simulink model "Optical_Movement_Detection_PAR"  (Simulink 7.5)
settings: Solver=ode45  StartTime=0.0  StopTime=inf  RelTol=1e-3
values from neighbouring files (symbols this model uses):
  D = 1    [Copter_Animation.m]
  HSE_Bottom_1 = imresize(imread('D:\GoogleMapsBilder\PAR\HSE_Bottom_1.jpg'), 1)    [TESTS_Optical_Flow_Scenarios.m]
undefined symbols (not defined in the file or in its folder): fspecial, Kanade, Low, Lucas, Rec, SDTV
libraries: simulink x13, dspobslib x10, vipgeotforms x3, vipanalysis x3, dspstat3 x3, dspmtrx3 x2, dspsigops x2, vipconversions x1, dspswit3 x1, vipsrcs x1, viptextngfix x1, vipsnks x1
(part 1 of 2)
settings Model: Creator=roczit00  LastModifiedBy=Anonymos
settings DataIOCC: SaveOutput=off  DSMLogging=off  SaveTime=off
settings DebuggingCC: AlgebraicLoopMsg=none  SolverPrmCheckMsg=none  UnconnectedInputMsg=none  UnconnectedOutputMsg=none  UnconnectedLineMsg=none  StrictBusMsg=Warning

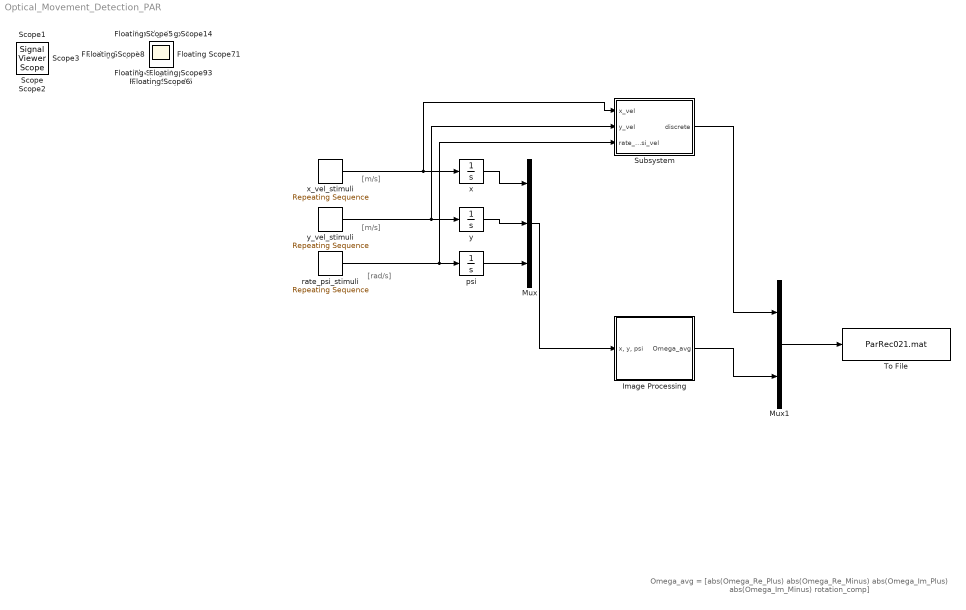
== system Optical_Movement_Detection_PAR ==
  note: [m/s]
  note: [m/s]
  note: [rad/s]
  note: Omega_avg = [abs(Omega_Re_Plus) abs(Omega_Re_Minus) abs(Omega_Im_Plus) abs(Omega_Im_Minus) rotation_comp]
  Image Processing : Subsystem  mask{Ts_Opt=10, Cam_Img_Dim=[100,100], Env_Orig=[2144 1424], Block_Matching_Size=[31,31], Block_Matching_Overlap=[0 0], Block_Matching_Max_Disp=[7 7], Omega_avg_Gain=1/1000, load_cmd=HSE_Bottom_1}
      mask prompts: Ts_Opt "Camera's frames per second (1/SampleTime):"; Cam_Img_Dim "Cameras size of the synthetic image [R C]:"; Env_Orig "Initial image center of environment [R C]:"; Block_Matching_Size "Block size of optical flow block matching algorithm [heigh width]"; Block_Matching_Overlap "Block Overlap [R C] :"; Block_Matching_Max_Disp "Maximum displacement [R C]:"; Omega_avg_Gain "Gain of detected velocity vector"; load_cmd "Load Cmd"
      mask init:
      | set_param(gcb,'MaskSelfModifiable','on')
      mask TabNameString: General,General,General,Block Matching,Block Matching,Block Matching,Block Matching,General
  Mux : Mux  Inputs=3
  Mux1 : Mux  Inputs=2
  Subsystem : Subsystem  mask{In_Val_Sample_Time=0.01}
      mask prompts: In_Val_Sample_Time "Sample time"
  To File : ToFile  Filename=ParRec021.mat  MatrixName=Tfile
  psi : Integrator
  rate_psi_stimuli : simulink/Sources/Repeating Sequence  SystemSampleTime=-1  rep_seq_t=[0,10]  rep_seq_y=[0,0]
  x : Integrator
  x_vel_stimuli : simulink/Sources/Repeating Sequence  SystemSampleTime=-1  rep_seq_t=[0,1]  rep_seq_y=[0,0.5]
  y : Integrator
  y_vel_stimuli : simulink/Sources/Repeating Sequence  SystemSampleTime=-1  rep_seq_t=[0,10]  rep_seq_y=[0,0]
  Floating Scope{,1..15} (16 alike) : Scope
      Floating Scope settings: Floating=on  YMin=-40  YMax=90
      Floating Scope1 settings: Floating=on
      Floating Scope10 settings: Floating=on  SaveName=ScopeData12
      Floating Scope11 settings: Floating=on  SaveName=ScopeData13
      Floating Scope12 settings: Floating=on  YMin=-2500  YMax=27500  SaveName=ScopeData14
      Floating Scope13 settings: Floating=on  YMin=3  YMax=7  SaveName=ScopeData15
      Floating Scope14 settings: Floating=on  SaveName=ScopeData16
      Floating Scope15 settings: Floating=on  SaveName=ScopeData17
      Floating Scope2 settings: Floating=on  YMin=-6000  YMax=2500  SaveName=ScopeData2
      Floating Scope3 settings: Floating=on  SaveName=ScopeData3
      Floating Scope4 settings: Floating=on  SaveName=ScopeData4
      Floating Scope5 settings: Floating=on  YMin=-0.7  YMax=0.8  SaveName=ScopeData5
      Floating Scope6 settings: Floating=on  YMin=-1  YMax=1  SaveName=ScopeData6
      Floating Scope7 settings: Floating=on  YMin=-15  YMax=10  SaveName=ScopeData7
      Floating Scope8 settings: Floating=on  YMax=45  SaveName=ScopeData10
      Floating Scope9 settings: Floating=on  YMin=-7  YMax=9  SaveName=ScopeData11
  Scope{,1..3} (4 alike) : SignalViewerScope  IOType=viewer  RefreshTime=0.035000
      Scope settings: YMin=-0.01  YMax=0.1
      Scope2 settings: SaveName=ScopeData2
      Scope3 settings: SaveName=ScopeData3
  wires:
  Mux/1 -> Image Processing/1("x, y, psi")
  y_vel_stimuli/1 -> y/1, Subsystem/2(y_vel)
  x_vel_stimuli/1 -> x/1, Subsystem/1(x_vel)
  rate_psi_stimuli/1 -> psi/1, Subsystem/3(rate_psi_vel)
  psi/1 -> Mux/3
  x/1 -> Mux/1
  y/1 -> Mux/2
  Mux1/1 -> To File/1
  Image Processing/1(Omega_avg) -> Mux1/2
  Subsystem/1(discrete) -> Mux1/1

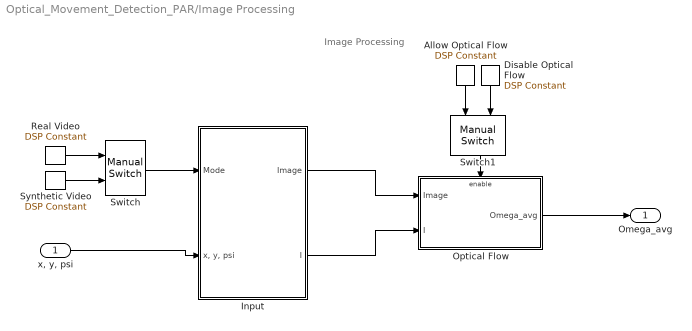
== system Optical_Movement_Detection_PAR/Image Processing ==
  note: Image Processing
  "x, y, psi" : Inport
  Allow Optical Flow : dspobslib/DSP Constant  SystemSampleTime=-1  Value=1  SampleMode=Discrete  discreteOutput=Sample-based  continuousOutput=Sample-based  sampTime=inf  framePeriod=2  dataType=boolean  isSigned=on  wordLen=16  udDataType=sfix(16)  fracBitsMode=Best precision  numFracBits=15  InterpretAs1D=-inf  Ts=-inf  FramebasedOutput=-inf
  Disable Optical Flow : dspobslib/DSP Constant  SystemSampleTime=-1  Value=0  SampleMode=Discrete  discreteOutput=Sample-based  continuousOutput=Sample-based  sampTime=inf  framePeriod=2  dataType=boolean  isSigned=on  wordLen=16  udDataType=sfix(16)  fracBitsMode=Best precision  numFracBits=15  InterpretAs1D=-inf  Ts=-inf  FramebasedOutput=-inf
  Input : Subsystem
      mask init:
      | set_param(gcb,'MaskSelfModifiable','on')
  Optical Flow : Subsystem
  Real Video : dspobslib/DSP Constant  SystemSampleTime=-1  Value=0  SampleMode=Discrete  discreteOutput=Sample-based  continuousOutput=Sample-based  sampTime=inf  framePeriod=2  dataType=boolean  isSigned=on  wordLen=16  udDataType=sfix(16)  fracBitsMode=Best precision  numFracBits=15  InterpretAs1D=-inf  Ts=-inf  FramebasedOutput=-inf
  Switch : simulink/Signal Routing/Manual Switch  SystemSampleTime=-1  sw=0  action=0  varsize=off
  Switch1 : simulink/Signal Routing/Manual Switch  SystemSampleTime=-1  sw=1  action=0  varsize=off
  Synthetic Video : dspobslib/DSP Constant  SystemSampleTime=-1  Value=1  SampleMode=Discrete  discreteOutput=Sample-based  continuousOutput=Sample-based  sampTime=inf  framePeriod=2  dataType=boolean  isSigned=on  wordLen=16  udDataType=sfix(16)  fracBitsMode=Best precision  numFracBits=15  InterpretAs1D=-inf  Ts=-inf  FramebasedOutput=-inf
  Omega_avg : Outport
  wires:
  Real Video/1 -> Switch/1
  Synthetic Video/1 -> Switch/2
  Switch/1 -> Input/1(Mode)
  "x, y, psi"/1 -> Input/2("x, y, psi")
  Input/1(Image) -> Optical Flow/1(Image)
  Input/2(I) -> Optical Flow/2(I)
  Allow Optical Flow/1 -> Switch1/1
  Disable Optical Flow/1 -> Switch1/2
  Optical Flow/1(Omega_avg) -> Omega_avg/1
  Switch1/1 -> Optical Flow/Enable

== system Optical_Movement_Detection_PAR/Subsystem ==
  note: discrete [x_vel_d y_vel_d rate_psi_vel_d]
  x_vel : Inport
  y_vel : Inport  Port=2
  rate_psi_vel : Inport  Port=3
  Mux3 : Mux  Inputs=3
  Zero-Order Hold2 : ZeroOrderHold  SampleTime=In_Val_Sample_Time
  Zero-Order Hold3 : ZeroOrderHold  SampleTime=In_Val_Sample_Time
  Zero-Order Hold4 : ZeroOrderHold  SampleTime=In_Val_Sample_Time
  discrete : Outport
  wires:
  Zero-Order Hold2/1 -> Mux3/1
  Zero-Order Hold3/1 -> Mux3/2
  Zero-Order Hold4/1 -> Mux3/3
  x_vel/1 -> Zero-Order Hold2/1
  y_vel/1 -> Zero-Order Hold3/1
  rate_psi_vel/1 -> Zero-Order Hold4/1
  Mux3/1 -> discrete/1

== system Optical_Movement_Detection_PAR/Image Processing/Input ==
  Mode : Inport  OutDataType=sfix(16)  OutScaling=2^0
  "x, y, psi" : Inport  Port=2  OutDataType=sfix(16)  OutScaling=2^0
  Color Space  Conversion : vipconversions/Color Space  Conversion  conversion=Obsolete  conversionActive=R'G'B' to intensity  wp_str=D65  rec=Rec. 601 (SDTV)  sys=1125/60/2:1  imagePorts=One multidimensional signal
  Synthetic Video Generation : Subsystem  mask(Synthetic Video Generation){dimen=Cam_Img_Dim, origin=Env_Orig, velocity=[100 100], varVelocity=[100 100], varCorner=[100 100], rotation=100, varRotation=100}
      mask prompts: dimen "Size of the synthetic image:"; origin "Initial image center:"; varVelocity "Variance of velocity:"; varCorner "Variance of corner location:"; rotation "Rotation speed (in degrees):"; varRotation "Variation of rotation (in degrees):"
      mask help: Generates a synthetic video.
  Zero-Order Hold1 : ZeroOrderHold  SampleTime=1/Ts_Opt
  Image : Outport
  I : Outport  Port=2
  wires:
  Mode/1 -> Synthetic Video Generation/Enable
  Color Space  Conversion/1 -> I/1
  Synthetic Video Generation/1(Image) -> Color Space  Conversion/1, Image/1
  "x, y, psi"/1 -> Zero-Order Hold1/1
  Zero-Order Hold1/1 -> Synthetic Video Generation/1("x, y, psi")

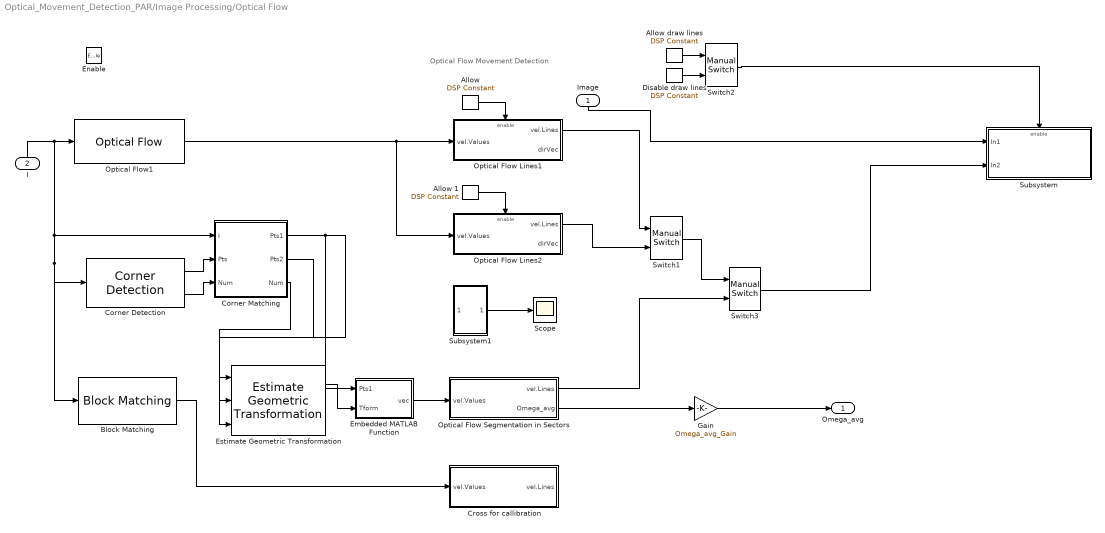
== system Optical_Movement_Detection_PAR/Image Processing/Optical Flow ==
  note: Optical Flow Movement Detection
  Image : Inport
  I : Inport  Port=2
  Enable : EnablePort  PropagateVarSize=During execution
  "Allow " : dspobslib/DSP Constant  SystemSampleTime=-1  Value=0  SampleMode=Discrete  discreteOutput=Sample-based  continuousOutput=Sample-based  sampTime=inf  framePeriod=2  dataType=boolean  isSigned=on  wordLen=16  udDataType=sfix(16)  fracBitsMode=Best precision  numFracBits=15  InterpretAs1D=-inf  Ts=-inf  FramebasedOutput=-inf
  Allow 1 : dspobslib/DSP Constant  SystemSampleTime=-1  Value=0  SampleMode=Discrete  discreteOutput=Sample-based  continuousOutput=Sample-based  sampTime=inf  framePeriod=2  dataType=boolean  isSigned=on  wordLen=16  udDataType=sfix(16)  fracBitsMode=Best precision  numFracBits=15  InterpretAs1D=-inf  Ts=-inf  FramebasedOutput=-inf
  Allow draw lines : dspobslib/DSP Constant  SystemSampleTime=-1  Value=1  SampleMode=Discrete  discreteOutput=Sample-based  continuousOutput=Sample-based  sampTime=inf  framePeriod=2  dataType=boolean  isSigned=on  wordLen=16  udDataType=sfix(16)  fracBitsMode=Best precision  numFracBits=15  InterpretAs1D=-inf  Ts=-inf  FramebasedOutput=-inf
  Block Matching : vipanalysis/Block Matching  DialogController=vipDDGCreate  DialogControllerArgs=DataTag3  SystemSampleTime=-1  which2img=Current frame and N-th frame back  N=1  searchMethod=Exhaustive  blockSize=Block_Matching_Size  overlapping=Block_Matching_Overlap  maxDisplacement=Block_Matching_Max_Disp  matchCriteria=Mean absolute difference (MAD)  outVelForm=Horizontal and vertical components in complex form  outputMode=Binary point scaling  outputWordLength=32  outputFracLength=0  accumMode=Binary point scaling  accumWordLength=64  accumFracLength=0  prodOutputMode=Binary point scaling  prodOutputWordLength=32  prodOutputFracLength=0  roundingMode=Ceiling  overflowMode=off
      link override Delay: dly_unit=Frames  delay=N
  Corner Detection : vipanalysis/Corner Detection  DialogController=vipDDGCreate  DialogControllerArgs=DataTag4  SystemSampleTime=-1  method=Local intensity comparison (Rosen & Drummond)  factor=0.04  filter=fspecial('gaussian', [1 5], 1.5)  thrInten=0.1  thrAngle=157.5  output=Corner location  outputInUse=Corner location  maxNum=75  thrMetric=0.001  neighborSize=[21 21]  isOutVarDim=on  accumMode=Binary point scaling  accumWordLength=32  accumFracLength=0  prodOutputMode=Binary point scaling  prodOutputWordLength=32  prodOutputFracLength=0  memoryMode=Binary point scaling  memoryWordLength=32  memoryFracLength=0  firstCoeffMode=Specify word length  firstCoeffWordLength=16  firstCoeffFracLength=16  roundingMode=Floor  overflowMode=off
  Corner Matching : Subsystem  mask(Corner Matching){winLen=9, maxNum=75, threshold=81}
      mask prompts: winLen "Block size used in corner matching:"; maxNum "Maximum number of points:"; threshold "Maximum feature difference for matching points:"
      mask help: Find out matching corners in the current and previous video frames.
  Cross for callibration : Subsystem  mask(Optical Flow Lines){scaleFactor=10}
      mask prompts: scaleFactor "Motion vector gain:"
      mask help: Generates the coordinate points of optical flow lines.
      mask Help: Generates the coordinate points of optical flow lines. Look under its mask to see the implementation details.
  Disable draw lines : dspobslib/DSP Constant  SystemSampleTime=-1  Value=0  SampleMode=Discrete  discreteOutput=Sample-based  continuousOutput=Sample-based  sampTime=inf  framePeriod=2  dataType=boolean  isSigned=on  wordLen=16  udDataType=sfix(16)  fracBitsMode=Best precision  numFracBits=15  InterpretAs1D=-inf  Ts=-inf  FramebasedOutput=-inf
  Embedded MATLAB Function : Stateflow chart  TreatAsAtomicUnit=on
  Estimate Geometric Transformation : vipgeotforms/Estimate Geometric Transformation  DialogController=vipDDGCreate  DialogControllerArgs=DataTag7  tformType=Projective  isRandomSampling=on  algMethod=Random Sample Consensus (RANSAC)  numMethod=Desired confidence  isStopSampling=on  percentStop=75  distanceAlg=1  distanceGeo=1.5  sampleNum=500  maxSampleNum=500  desiredConfidence=99  isRefineTForm=on  isOutputInlier=on  outDT4IntInput=Single  outDT4IntInputActive=Single  isVarSizeAllowed=on  isReleaseMode=on
  Gain : Gain  Gain=Omega_avg_Gain  ParameterDataType=fixdt(1, 16)  ParameterScaling=2^0  OutDataType=fixdt(1, 16)  OutScaling=2^0
  Optical Flow Lines1 : Subsystem  mask(Optical Flow Lines){scaleFactor=0.0008}
      mask prompts: scaleFactor "Motion vector gain:"
      mask help: Generates the coordinate points of optical flow lines.
      mask Help: Generates the coordinate points of optical flow lines. Look under its mask to see the implementation details.
  Optical Flow Lines2 : Subsystem  mask(Optical Flow Lines){scaleFactor=5}
      mask prompts: scaleFactor "Motion vector gain:"
      mask help: Generates the coordinate points of optical flow lines.
      mask Help: Generates the coordinate points of optical flow lines. Look under its mask to see the implementation details.
  Optical Flow Segmentation in Sectors : Subsystem  mask(Optical Flow Lines){scaleFactor=10}
      mask prompts: scaleFactor "Motion vector gain:"
      mask help: Generates the coordinate points of optical flow lines.
      mask Help: Generates the coordinate points of optical flow lines. Look under its mask to see the implementation details.
  Optical Flow1 : vipanalysis/Optical Flow  DialogController=vipDDGCreate  DialogControllerArgs=DataTag8  SystemSampleTime=-1  method=Lucas-Kanade  gradMethod=Derivative of Gaussian  which2img=Current frame and N-th frame back  N=1  outVelForm=Horizontal and vertical components in complex form  lambda=1  stop_criteria=When maximum number of iterations is reached  maxAllowAbsDiff=eps  maxIter=10  numInports=3  sigmaS=1.5  sigmaW=1  eigTh=0.0039  discardNormalFlow=on  outputCurrentImage=off  prodOutputMode=Binary point scaling  prodOutputWordLength=32  prodOutputFracLength=20  outputMode=Binary point scaling  outputWordLength=32  outputFracLength=20  roundingMode=Nearest  overflowMode=on
  Scope : Scope
      settings: YMin=0  YMax=10  SaveName=ScopeData8
  Subsystem : Subsystem
  Subsystem1 : Subsystem
  Switch1 : simulink/Signal Routing/Manual Switch  SystemSampleTime=-1  sw=0  action=0  varsize=off
  Switch2 : simulink/Signal Routing/Manual Switch  SystemSampleTime=-1  sw=1  action=0  varsize=off
  Switch3 : simulink/Signal Routing/Manual Switch  SystemSampleTime=-1  sw=0  action=0  varsize=on
  Omega_avg : Outport
  wires:
  Image/1 -> Subsystem/1(In1)
  I/1 -> Optical Flow1/1, Corner Matching/1(I), Block Matching/1, Corner Detection/1
  Allow draw lines/1 -> Switch2/1
  Disable draw lines/1 -> Switch2/2
  Switch2/1 -> Subsystem/Enable
  Subsystem1/1(angle) -> Scope/1
  Optical Flow Lines2/1(vel.Lines) -> Switch1/2
  Optical Flow Lines1/1(vel.Lines) -> Switch1/1
  Optical Flow1/1 -> Optical Flow Lines1/1(vel.Values), Optical Flow Lines2/1(vel.Values)
  Optical Flow Segmentation in Sectors/1(vel.Lines) -> Switch3/2
  Switch1/1 -> Switch3/1
  "Allow "/1 -> Optical Flow Lines1/Enable
  Allow 1/1 -> Optical Flow Lines2/Enable
  Optical Flow Segmentation in Sectors/2(Omega_avg) -> Gain/1
  Block Matching/1 -> Cross for callibration/1(vel.Values)
  Switch3/1 -> Subsystem/2(In2)
  Gain/1 -> Omega_avg/1
  Corner Detection/1 -> Corner Matching/2(Pts)
  Corner Detection/2 -> Corner Matching/3(Num)
  Embedded MATLAB Function/1(vec) -> Optical Flow Segmentation in Sectors/1(vel.Values)
  Corner Matching/1(Pts1) -> Estimate Geometric Transformation/1, Embedded MATLAB Function/1(Pts1)
  Corner Matching/2(Pts2) -> Estimate Geometric Transformation/2
  Corner Matching/3("Num ") -> Estimate Geometric Transformation/3
  Estimate Geometric Transformation/1 -> Embedded MATLAB Function/2(Tform)

== system Optical_Movement_Detection_PAR/Image Processing/Input/Synthetic Video Generation ==
  "x, y, psi" : Inport  OutDataType=sfix(16)  OutScaling=2^0
  Enable : EnablePort  PropagateVarSize=During execution
  N-Sample Enable : dspswit3/N-Sample Enable  N=1  ActiveLevel=Low (0)  reset=off  TriggerType=Rising edge  Ts=-1  DataType=Logical
  Read Image : Subsystem
      settings: AttributesFormatString=Load image only at the beginning of simulation
  Synthesize Video : Subsystem  mask{dimen=dimen, origin=origin, velocity=velocity, varVelocity=varVelocity, varCorner=varCorner, rotation=rotation, varRotation=varRotation}
      mask prompts: dimen "Size of the synthetic image:"; origin "Initial image center:"; varVelocity "Variance of velocity:"; varCorner "Variance of corner location:"; rotation "Rotation speed:"; varRotation "Variation of rotation:"
  Image : Outport
  Reset : Outport  Port=2  InitialOutput=1
  wires:
  Read Image/2(Size) -> Synthesize Video/2(Size)
  Read Image/1(Image) -> Synthesize Video/1("Image ")
  N-Sample Enable/1 -> Read Image/Enable
  Synthesize Video/2(Reset) -> Reset/1
  Synthesize Video/1(Image) -> Image/1
  "x, y, psi"/1 -> Synthesize Video/3("x, y, psi")

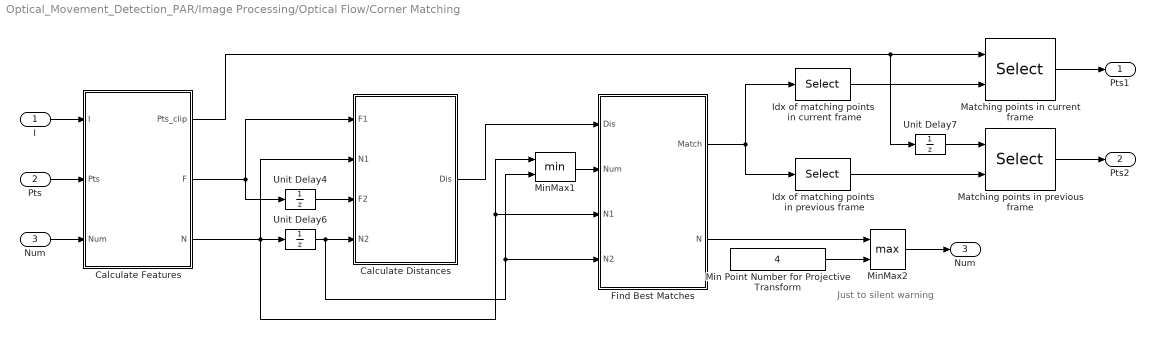
== system Optical_Movement_Detection_PAR/Image Processing/Optical Flow/Corner Matching ==
  note: Just to
      | silent warning
  I : Inport  OutDataType=sfix(16)  OutScaling=2^0
  Pts : Inport  Port=2  OutDataType=sfix(16)  OutScaling=2^0
  Num : Inport  Port=3  OutDataType=sfix(16)  OutScaling=2^0
  Calculate Distances : Subsystem  TreatAsAtomicUnit=on  mask{maxNum=maxNum}
      mask prompts: maxNum "Maximum data number:"
      settings: AttributesFormatString=between features.
  Calculate Features : Subsystem  TreatAsAtomicUnit=on  mask{winLen=winLen, maxNum=maxNum}
      mask prompts: winLen "Neighborhood size:"; maxNum "Maximum number of features:"
  Find Best Matches : Subsystem  TreatAsAtomicUnit=on  mask{maxNum=maxNum, threshold=threshold}
      mask prompts: maxNum "Maximum data number:"
      settings: AttributesFormatString=between the features\nin the current and previous frames
  Idx of matching points  in current frame : Selector  NumberOfDimensions=2  IndexMode=Zero-based  InputPortWidth=2  IndexOptions=Index vector (dialog),Select all  Indices=0,1  OutputSizes=1,1
  Idx of matching points  in previous frame : Selector  NumberOfDimensions=2  IndexMode=Zero-based  InputPortWidth=2  IndexOptions=Index vector (dialog),Select all  Indices=1,1  OutputSizes=1,1
  Matching points in current frame : Selector  NumberOfDimensions=2  IndexMode=Zero-based  InputPortWidth=2  IndexOptions=Select all,Index vector (port)  Indices=0,1  OutputSizes=1,1
  Matching points in previous frame : Selector  NumberOfDimensions=2  IndexMode=Zero-based  InputPortWidth=2  IndexOptions=Select all,Index vector (port)  Indices=0,1  OutputSizes=1,1
  Min Point Number for Projective Transform : Constant  Value=4  OutDataType=sfix(16)  OutScaling=2^0  OutDataTypeStr=Inherit: Inherit via back propagation
  MinMax1 : MinMax  Inputs=2  OutDataType=sfix(16)  OutScaling=2^0
  MinMax2 : MinMax  Function=max  Inputs=2  OutDataType=sfix(16)  OutScaling=2^0  OutDataTypeStr=Inherit: Inherit via back propagation
  Unit Delay4 : UnitDelay  SampleTime=-1
  Unit Delay6 : UnitDelay  SampleTime=-1
  Unit Delay7 : UnitDelay  SampleTime=-1
  Pts1 : Outport  OutDataType=sfix(16)  OutScaling=2^0
  Pts2 : Outport  Port=2  OutDataType=sfix(16)  OutScaling=2^0
  "Num " : Outport  Port=3  OutDataType=sfix(16)  OutScaling=2^0
  wires:
  Calculate Features/2(F) -> Calculate Distances/1(F1), Unit Delay4/1
  Calculate Features/3(N) -> Calculate Distances/2(N1), Unit Delay6/1, MinMax1/1, Find Best Matches/3(N1)
  Calculate Features/1(Pts_clip) -> Unit Delay7/1, Matching points in current frame/1
  Num/1 -> Calculate Features/3(Num)
  Unit Delay6/1 -> Calculate Distances/4(N2), MinMax1/2, Find Best Matches/4(N2)
  Unit Delay4/1 -> Calculate Distances/3(F2)
  Matching points in previous frame/1 -> Pts2/1
  Matching points in current frame/1 -> Pts1/1
  Unit Delay7/1 -> Matching points in previous frame/1
  Idx of matching points  in current frame/1 -> Matching points in current frame/2
  Idx of matching points  in previous frame/1 -> Matching points in previous frame/2
  Find Best Matches/1(Match) -> Idx of matching points  in previous frame/1, Idx of matching points  in current frame/1
  Calculate Distances/1(Dis) -> Find Best Matches/1(Dis)
  I/1 -> Calculate Features/1(I)
  Pts/1 -> Calculate Features/2(Pts)
  Min Point Number for Projective Transform/1 -> MinMax2/2
  Find Best Matches/2(N) -> MinMax2/1
  MinMax2/1 -> "Num "/1
  MinMax1/1 -> Find Best Matches/2(Num)

== system Optical_Movement_Detection_PAR/Image Processing/Optical Flow/Cross for callibration ==
  vel.Values : Inport  OutDataType=sfix(16)  OutScaling=2^0
  " " : dspobslib/DSP Constant  SystemSampleTime=-1  Value=Cam_Img_Dim  SampleMode=Discrete  discreteOutput=Sample-based  continuousOutput=Sample-based  sampTime=inf  framePeriod=2  dataType=double  isSigned=on  wordLen=16  udDataType=sfix(16)  fracBitsMode=Best precision  numFracBits=15  InterpretAs1D=-inf  Ts=-inf  FramebasedOutput=-inf
  Optical Flow Lines1 : Stateflow chart  TreatAsAtomicUnit=on
  vel.Lines : Outport  OutDataType=sfix(16)  OutScaling=2^0
  wires:
  Optical Flow Lines1/1(vel_Lines) -> vel.Lines/1
  vel.Values/1 -> Optical Flow Lines1/1(vel_Values)
  " "/1 -> Optical Flow Lines1/2(Cam_Img_Dim)

== system Optical_Movement_Detection_PAR/Image Processing/Optical Flow/Optical Flow Lines1 ==
  vel.Values : Inport  OutDataType=sfix(16)  OutScaling=2^0
  Enable : EnablePort  PropagateVarSize=During execution
  Optical Flow Lines1 : Stateflow chart  TreatAsAtomicUnit=on
  vel.Lines : Outport  OutDataType=sfix(16)  OutScaling=2^0
  dirVec : Outport  Port=2  OutDataType=sfix(16)  OutScaling=2^0
  wires:
  Optical Flow Lines1/1(vel_Lines) -> vel.Lines/1
  vel.Values/1 -> Optical Flow Lines1/1(vel_Values)
  Optical Flow Lines1/2(dir_Vec) -> dirVec/1

== system Optical_Movement_Detection_PAR/Image Processing/Optical Flow/Optical Flow Lines2 ==
  vel.Values : Inport  OutDataType=sfix(16)  OutScaling=2^0
  Enable : EnablePort  PropagateVarSize=During execution
  Optical Flow Lines1 : Stateflow chart  TreatAsAtomicUnit=on
  vel.Lines : Outport  OutDataType=sfix(16)  OutScaling=2^0
  dirVec : Outport  Port=2  OutDataType=sfix(16)  OutScaling=2^0
  wires:
  Optical Flow Lines1/1(vel_Lines) -> vel.Lines/1
  vel.Values/1 -> Optical Flow Lines1/1(vel_Values)
  Optical Flow Lines1/2(dir_Vec) -> dirVec/1

== system Optical_Movement_Detection_PAR/Image Processing/Optical Flow/Optical Flow Segmentation in Sectors ==
  note: Omega_avg = [abs(Omega_Re_Plus) abs(Omega_Re_Minus) abs(Omega_Im_Plus) abs(Omega_Im_Minus) rotation_comp]
  vel.Values : Inport  OutDataType=sfix(16)  OutScaling=2^0
  " " : dspobslib/DSP Constant  SystemSampleTime=-1  Value=Cam_Img_Dim  SampleMode=Discrete  discreteOutput=Sample-based  continuousOutput=Sample-based  sampTime=inf  framePeriod=2  dataType=double  isSigned=on  wordLen=16  udDataType=sfix(16)  fracBitsMode=Best precision  numFracBits=15  InterpretAs1D=-inf  Ts=-inf  FramebasedOutput=-inf
  Optical Flow Lines1 : Stateflow chart  TreatAsAtomicUnit=on
  vel.Lines : Outport  OutDataType=sfix(16)  OutScaling=2^0
  Omega_avg : Outport  Port=2  OutDataType=sfix(16)  OutScaling=2^0
  wires:
  Optical Flow Lines1/1(vel_Lines) -> vel.Lines/1
  vel.Values/1 -> Optical Flow Lines1/1(vel_Values)
  Optical Flow Lines1/2(Omega_avg) -> Omega_avg/1
  " "/1 -> Optical Flow Lines1/2(Cam_Img_Dim)

== system Optical_Movement_Detection_PAR/Image Processing/Optical Flow/Subsystem ==
  In1 : Inport
  In2 : Inport  Port=2
  Enable : EnablePort  PropagateVarSize=During execution
  Draw Shapes1 : viptextngfix/Draw Shapes  DialogController=vipDDGCreate  DialogControllerArgs=DataTag9  shape=Lines  fill=off  fillClrSource=Specify via dialog  display=User-specified value  intensity=200  color=[255 255 0]  opacity=0.6  viewport=Entire image  antialiasing=off  inType=Obsolete  imagePorts=One multidimensional signal  prodOutputMode=Binary point scaling  prodOutputWordLength=32  prodOutputFracLength=14  memoryMode=Specify word length  memoryWordLength=16  memoryFracLength=15  roundingMode=Floor  overflowMode=off
  To Video Display : vipsnks/To Video Display  DialogControllerArgs=DataTag10  inputType=Obsolete  imagePorts=One multidimensional signal  OutputDevice=On-screen video monitor  fullScreen=off  videoWindowX=527  videoWindowY=141  saveWindowSize=off  videoWindowWidth=116  videoWindowHeight=100  dataOrg=Column-major  openAtMdlStart=on  isWindowOpen=on
  wires:
  Draw Shapes1/1 -> To Video Display/1
  In1/1 -> Draw Shapes1/1
  In2/1 -> Draw Shapes1/2

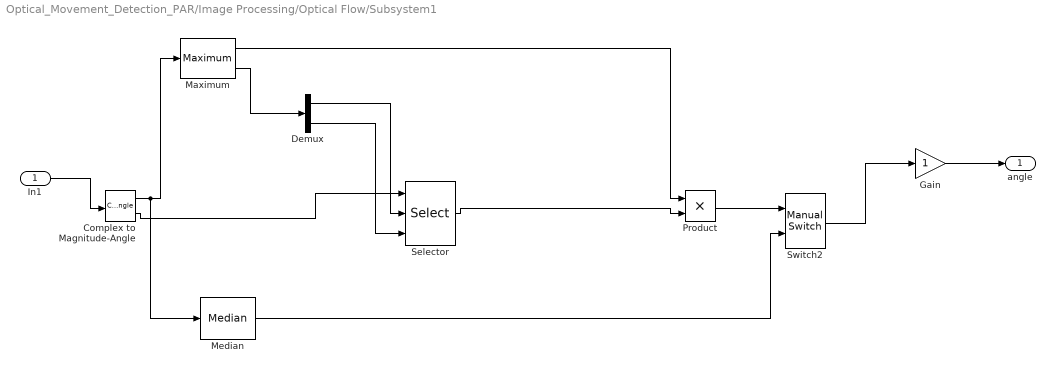
== system Optical_Movement_Detection_PAR/Image Processing/Optical Flow/Subsystem1 ==
  In1 : Inport
  Complex to Magnitude-Angle : ComplexToMagnitudeAngle
  Demux : Demux  Outputs=2
  Gain : Gain  ParameterDataType=fixdt(1, 16)  ParameterScaling=2^0  OutDataType=fixdt(1, 16)  OutScaling=2^0
  Maximum : dspstat3/Maximum  DialogController=dspDDGCreate  DialogControllerArgs=DataTag11  fcn=Value and Index  reset=None  indexBase=One  operateOver=Entire input  Dimension=1  colComp=off  operation=maximum  roiEnable=off  roiType=Lines  roiPortion=Entire ROI  roiOutput=Individual statistics for each ROI  roiFlag=off  accumDataTypeStr=Inherit: Same as product output  accumLastDataTypeStr=Inherit: Same as product output  roundingMode=Floor  overflowMode=on
  Median : dspstat3/Median  DialogController=dspDDGCreate  DialogControllerArgs=DataTag12  sortAlg=Quick sort  directionMode=Entire input  dimension=2  treatSBRowAsCol=on  outputMin=[]  outputMax=[]  accumDataTypeStr=Inherit: Same as product output  accumLastDataTypeStr=Inherit: Same as product output  roundingMode=Ceiling  overflowMode=on
      settings: allowOverrides=off
  Product : Product  OutDataType=fixdt(1, 16)  OutScaling=2^0  RndMeth=Zero
  Selector : Selector  NumberOfDimensions=2  InputPortWidth=3  IndexOptions=Index vector (port),Index vector (port)  Indices=[0],1  OutputSizes=1,1
  Switch2 : simulink/Signal Routing/Manual Switch  SystemSampleTime=-1  sw=0  action=0  varsize=off
  angle : Outport  OutDataType=fixdt(1, 16)  OutScaling=2^0
  wires:
  In1/1 -> Complex to Magnitude-Angle/1
  Complex to Magnitude-Angle/1 -> Maximum/1, Median/1
  Complex to Magnitude-Angle/2 -> Selector/1
  Demux/1 -> Selector/2
  Gain/1 -> angle/1
  Demux/2 -> Selector/3
  Maximum/1 -> Product/1
  Selector/1 -> Product/2
  Maximum/2 -> Demux/1
  Product/1 -> Switch2/1
  Median/1 -> Switch2/2
  Switch2/1 -> Gain/1

== system Optical_Movement_Detection_PAR/Image Processing/Input/Synthetic Video Generation/Read Image ==
  Enable : EnablePort  PropagateVarSize=During execution
  Image From Workspace : vipsrcs/Image From Workspace  Tag=vipblks_nd  SystemSampleTime=-1  ImageValue=load_cmd  Ts=inf  imagePorts=One multidimensional signal  ImageDataType=single  Signed=on  WordLength=16  sdImageDataType=sfix(16)  FractionLengthMode=User-defined  FractionLength=15  OutPortLabels=R|G|B
  Probe : Probe  ProbeWidth=off  ProbeSampleTime=off  ProbeComplexSignal=off  ProbeSignalDimensions=on  ProbeDimensionsDataType=single
  Image : Outport  InitialOutput=0
  Size : Outport  Port=2
  wires:
  Image From Workspace/1 -> Probe/1, Image/1
  Probe/1 -> Size/1

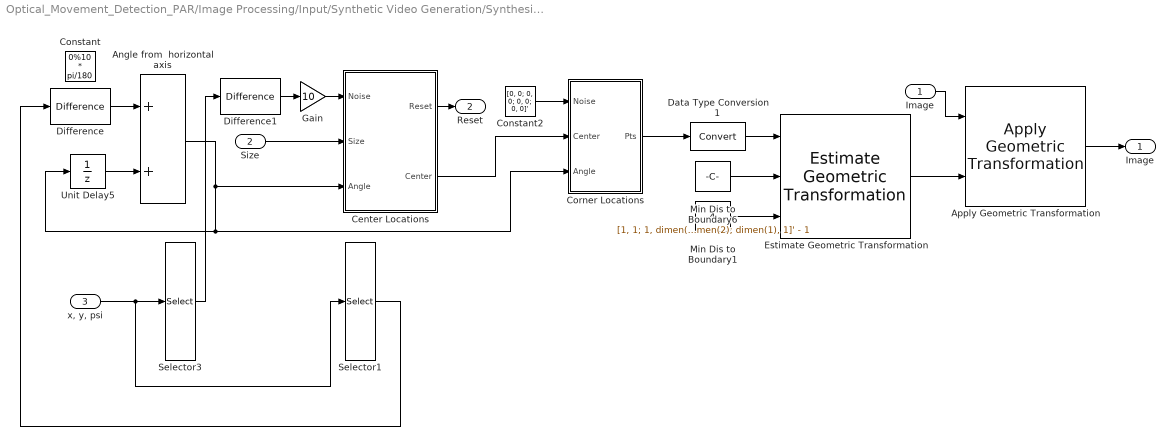
== system Optical_Movement_Detection_PAR/Image Processing/Input/Synthetic Video Generation/Synthesize Video ==
  "Image " : Inport  OutDataType=sfix(16)  OutScaling=2^0
  Size : Inport  Port=2  OutDataType=sfix(16)  OutScaling=2^0
  "x, y, psi" : Inport  Port=3  OutDataType=sfix(16)  OutScaling=2^0
  Angle from  horizontal axis : Sum  OutDataType=sfix(16)  OutScaling=2^-10
  Apply Geometric Transformation : vipgeotforms/Apply Geometric Transformation  DialogController=vipDDGCreate  DialogControllerArgs=DataTag0  tformSource=Input port  tformValue=[1 0 0; 0 1 0; 0 0 1]  approxProjectiveFlag=off  errorTolerance=1.0  roiMethod=Whole input image  roiSource=Specify via dialog  roiBBox=[0 0 128 256]  roiVertice=[0 0 10 12 20 22]  inputClipFlag=off  interpolationMethod=Bilinear  fillValue=0  viewPortMethod=Specify via dialog  outputSize=dimen  outputLoc=[0 0]  outputClipFlag=off
  Center Locations : Subsystem
  Constant : Constant  Value=0%10 * pi/180  OutDataType=fixdt(1, 16)  OutScaling=2^0
  Constant2 : Constant  Value=[0, 0; 0, 0; 0, 0; 0, 0]'  OutDataType=fixdt(1, 16)  OutScaling=2^0
  Corner Locations : Subsystem
  Data Type Conversion1 : DataTypeConversion  OutDataType=sfix(16)  OutScaling=2^0
  Difference : simulink/Discrete/Difference  SystemSampleTime=-1  ICPrevInput=0.0  OutMin=[]  OutMax=[]  OutDataType=fixdt(1, 16)  OutScaling=2^-10  DoSatur=off
  Difference1 : simulink/Discrete/Difference  SystemSampleTime=-1  ICPrevInput=0.0  OutMin=[]  OutMax=[]  OutDataType=fixdt(1, 16)  OutScaling=2^-10  DoSatur=off
  Estimate Geometric Transformation : vipgeotforms/Estimate Geometric Transformation  DialogController=vipDDGCreate  DialogControllerArgs=DataTag2  tformType=Projective  isRandomSampling=off  algMethod=Random Sample Consensus (RANSAC)  numMethod=Specified value  isStopSampling=off  percentStop=75  distanceAlg=1.5  distanceGeo=1.5  sampleNum=100  maxSampleNum=200  desiredConfidence=99  isRefineTForm=off  isOutputInlier=off  outDT4IntInput=Obsolete10a  outDT4IntInputActive=Single  isVarSizeAllowed=off  isReleaseMode=on
  Gain : Gain  Gain=10  ParameterDataType=fixdt(1, 16)  ParameterScaling=2^0  OutDataType=fixdt(1, 16)  OutScaling=2^0
  Min Dis to Boundary1 : Constant  Value=4  OutDataType=sfix(16)  OutScaling=2^0  OutDataTypeStr=Inherit: Inherit via back propagation
  Min Dis to Boundary6 : Constant  Value=[1, 1; 1, dimen(2); dimen(1), dimen(2); dimen(1), 1]' - 1  OutDataType=sfix(16)  OutScaling=2^0  OutDataTypeStr=Inherit: Inherit via back propagation
  Selector1 : Selector  InputPortWidth=3  IndexOptions=Index vector (dialog)  Indices=[3]  OutputSizes=1
  Selector3 : Selector  InputPortWidth=3  IndexOptions=Index vector (dialog)  Indices=[2 1]  OutputSizes=1
  Unit Delay5 : UnitDelay  X0=-pi/12  SampleTime=-1
  Image : Outport  OutDataType=sfix(16)  OutScaling=2^0
  Reset : Outport  Port=2  OutDataType=sfix(16)  OutScaling=2^0
  wires:
  Constant2/1 -> Corner Locations/1(Noise)
  Angle from  horizontal axis/1 -> Center Locations/3(Angle), Corner Locations/3(Angle), Unit Delay5/1
  Center Locations/1(Reset) -> Reset/1
  Size/1 -> Center Locations/2(Size)
  Min Dis to Boundary6/1 -> Estimate Geometric Transformation/2
  Min Dis to Boundary1/1 -> Estimate Geometric Transformation/3
  Data Type Conversion1/1 -> Estimate Geometric Transformation/1
  Estimate Geometric Transformation/1 -> Apply Geometric Transformation/2
  Corner Locations/1(Pts) -> Data Type Conversion1/1
  "x, y, psi"/1 -> Selector3/1, Selector1/1
  Center Locations/2(Center) -> Corner Locations/2(Center)
  "Image "/1 -> Apply Geometric Transformation/1
  Apply Geometric Transformation/1 -> Image/1
  Unit Delay5/1 -> Angle from  horizontal axis/2
  Selector1/1 -> Difference/1
  Selector3/1 -> Difference1/1
  Difference/1 -> Angle from  horizontal axis/1
  Difference1/1 -> Gain/1
  Gain/1 -> Center Locations/1(Noise)

== system Optical_Movement_Detection_PAR/Image Processing/Optical Flow/Corner Matching/Calculate Distances ==
  F1 : Inport  OutDataType=sfix(16)  OutScaling=2^0
  N1 : Inport  Port=2  OutDataType=sfix(16)  OutScaling=2^0
  F2 : Inport  Port=3  OutDataType=sfix(16)  OutScaling=2^0
  N2 : Inport  Port=4  OutDataType=sfix(16)  OutScaling=2^0
  For Iterator Subsystem : Subsystem  TreatAsAtomicUnit=on
  Initial Values1 : Constant  Value=maxNum  OutDataType=sfix(16)  OutScaling=2^0  OutDataTypeStr=Inherit: Inherit via back propagation  SampleTime=-1
  Initial Values2 : Constant  Value=maxNum  OutDataType=sfix(16)  OutScaling=2^0  OutDataTypeStr=Inherit: Inherit via back propagation  SampleTime=-1
  MinMax1 : MinMax  Inputs=2  OutDataType=sfix(16)  OutScaling=2^0
  MinMax2 : MinMax  Inputs=2  OutDataType=sfix(16)  OutScaling=2^0
  Dis : Outport  OutDataType=sfix(16)  OutScaling=2^0
  wires:
  MinMax2/1 -> For Iterator Subsystem/4(N2)
  F2/1 -> For Iterator Subsystem/3(F2)
  MinMax1/1 -> For Iterator Subsystem/2(N1)
  F1/1 -> For Iterator Subsystem/1(F1)
  For Iterator Subsystem/1(Dis) -> Dis/1
  N2/1 -> MinMax2/2
  Initial Values2/1 -> MinMax2/1
  N1/1 -> MinMax1/2
  Initial Values1/1 -> MinMax1/1

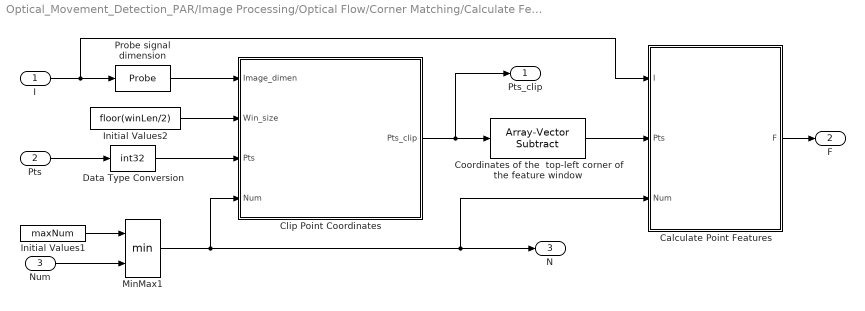
== system Optical_Movement_Detection_PAR/Image Processing/Optical Flow/Corner Matching/Calculate Features ==
  I : Inport  OutDataType=sfix(16)  OutScaling=2^0
  Pts : Inport  Port=2  OutDataType=sfix(16)  OutScaling=2^0
  Num : Inport  Port=3  OutDataType=sfix(16)  OutScaling=2^0
  Calculate Point Features : Subsystem
  Clip Point Coordinates : Subsystem
  Coordinates of the  top-left corner of the feature window : dspmtrx3/Array-Vector Subtract  DialogController=dspDDGCreate  DialogControllerArgs=DataTag5  Dimension=1  V_Source=Dialog parameter  V_VectFromMask=floor([winLen; winLen] / 2)  firstCoeffDataTypeStr=Inherit: Same word length as input  firstCoeffLastDataTypeStr=Inherit: Same word length as input  firstCoeffMin=[]  firstCoeffMax=[]  outputMin=[]  outputMax=[]  roundingMode=Floor  overflowMode=off
  Data Type Conversion : DataTypeConversion  OutDataTypeMode=int32  OutDataType=sfix(16)  OutScaling=2^0  OutDataTypeStr=int32
  Initial Values1 : Constant  Value=maxNum  OutDataType=sfix(16)  OutScaling=2^0  OutDataTypeStr=Inherit: Inherit via back propagation  SampleTime=-1
  Initial Values2 : Constant  Value=floor(winLen/2)  OutDataType=sfix(16)  OutScaling=2^0  OutDataTypeStr=Inherit: Inherit via back propagation  SampleTime=-1
  MinMax1 : MinMax  Inputs=2  OutDataType=sfix(16)  OutScaling=2^0
  Probe signal dimension : Probe  ProbeWidth=off  ProbeSampleTime=off  ProbeComplexSignal=off  ProbeSignalDimensions=on  ProbeDimensionsDataType=int32
  Pts_clip : Outport  OutDataType=sfix(16)  OutScaling=2^0
  F : Outport  Port=2  OutDataType=sfix(16)  OutScaling=2^0
  N : Outport  Port=3  OutDataType=sfix(16)  OutScaling=2^0
  wires:
  Data Type Conversion/1 -> Clip Point Coordinates/3(Pts)
  MinMax1/1 -> N/1, Calculate Point Features/3(Num), Clip Point Coordinates/4(Num)
  Coordinates of the  top-left corner of the feature window/1 -> Calculate Point Features/2(Pts)
  Clip Point Coordinates/1(Pts_clip) -> Coordinates of the  top-left corner of the feature window/1, Pts_clip/1
  Pts/1 -> Data Type Conversion/1
  Initial Values2/1 -> Clip Point Coordinates/2(Win_size)
  Probe signal dimension/1 -> Clip Point Coordinates/1(Image_dimen)
  I/1 -> Calculate Point Features/1(I), Probe signal dimension/1
  Initial Values1/1 -> MinMax1/1
  Num/1 -> MinMax1/2
  Calculate Point Features/1(F) -> F/1

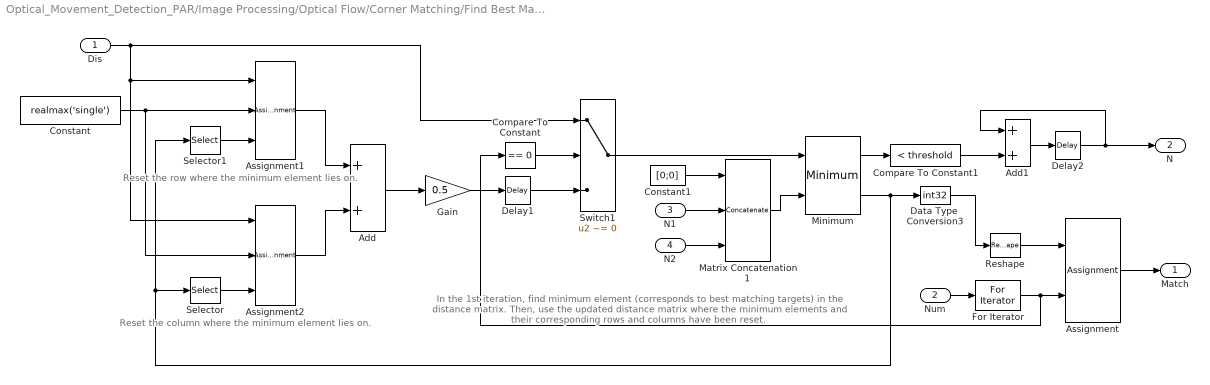
== system Optical_Movement_Detection_PAR/Image Processing/Optical Flow/Corner Matching/Find Best Matches ==
  note: In the 1st iteration, find minimum element (corresponds to
      | best matching targets) in the distance matrix. Then, use the
      | updated distance matrix where the minimum elements and
      | their  corresponding rows and columns have been reset.
  note: Reset the column where the
      | minimum element lies on.
  note: Reset the row where the
      | minimum element lies on.
  Dis : Inport  OutDataType=sfix(16)  OutScaling=2^0
  Num : Inport  Port=2  OutDataType=sfix(16)  OutScaling=2^0
  N1 : Inport  Port=3  OutDataType=sfix(16)  OutScaling=2^0
  N2 : Inport  Port=4  OutDataType=sfix(16)  OutScaling=2^0
  Add : Sum  OutDataType=sfix(16)  OutScaling=2^-10
  Add1 : Sum  OutDataTypeMode=int32  OutDataType=sfix(16)  OutScaling=2^-10  OutDataTypeStr=int32
  Assignment : Assignment  NumberOfDimensions=2  IndexMode=Zero-based  OutputInitialize=Specify size for each dimension in table  IndexOptions=Assign all,Index vector (port)  Indices=-1,-1  OutputSizes=2,maxNum
  Assignment1 : Assignment  NumberOfDimensions=2  IndexMode=Zero-based  IndexOptions=Index vector (port),Assign all  Indices=1,-1  OutputSizes=1,1
  Assignment2 : Assignment  NumberOfDimensions=2  IndexMode=Zero-based  IndexOptions=Assign all,Index vector (port)  Indices=-1,-1  OutputSizes=1,1
  Compare To Constant : simulink/Logic and Bit Operations/Compare To Constant  SystemSampleTime=-1  relop===  const=0  LogicOutDataTypeMode=boolean  ZeroCross=off
  Compare To Constant1 : simulink/Logic and Bit Operations/Compare To Constant  SystemSampleTime=-1  relop=<  const=threshold  LogicOutDataTypeMode=uint8  ZeroCross=off
  Constant : Constant  Value=realmax('single')  VectorParams1D=off  OutDataType=sfix(16)  OutScaling=2^0  OutDataTypeStr=Inherit: Inherit via back propagation
  Constant1 : Constant  Value=[0;0]  VectorParams1D=off  OutDataType=sfix(16)  OutScaling=2^0  OutDataTypeStr=Inherit: Inherit via back propagation
  Data Type  Conversion3 : DataTypeConversion  OutDataTypeMode=int32  OutDataType=sfix(16)  OutScaling=2^0  OutDataTypeStr=int32  SaturateOnIntegerOverflow=on  RndMeth=Zero
  Delay1 : dspsigops/Delay  dly_unit=Samples  delay=1  ic_detail=off  dif_ic_for_ch=off  dif_ic_for_dly=off  ic=0  reset_popup=None
  Delay2 : dspsigops/Delay  dly_unit=Samples  delay=1  ic_detail=off  dif_ic_for_ch=off  dif_ic_for_dly=off  ic=0  reset_popup=None
  For Iterator : ForIterator  ResetStates=reset  IterationSource=external  IterationLimit=expLaneNum  IndexMode=Zero-based
  Gain : Gain  Gain=0.5  ParameterDataType=sfix(16)  ParameterScaling=2^0  OutDataType=sfix(16)  OutScaling=2^0
  Matrix Concatenation1 : Concatenate  NumInputs=3  Mode=Multidimensional array
  Minimum : dspstat3/Minimum  DialogController=dspDDGCreate  DialogControllerArgs=DataTag6  fcn=Value and Index  reset=None  indexBase=Zero  operateOver=Entire input  Dimension=1  colComp=on  operation=minimum  roiEnable=on  roiType=Rectangles  roiPortion=Entire ROI  roiOutput=Individual statistics for each ROI  roiFlag=off  roundingMode=Floor  overflowMode=off
  Reshape : Reshape  OutputDimensionality=Column vector (2-D)
  Selector : Selector  IndexMode=Zero-based  InputPortWidth=2  IndexOptions=Index vector (dialog)  Indices=1  OutputSizes=1
  Selector1 : Selector  IndexMode=Zero-based  InputPortWidth=2  IndexOptions=Index vector (dialog)  Indices=0  OutputSizes=1
  Switch1 : Switch  Criteria=u2 ~= 0  OutDataType=sfix(16)  OutScaling=2^0
  Match : Outport  OutDataType=sfix(16)  OutScaling=2^0
  N : Outport  Port=2  OutDataType=sfix(16)  OutScaling=2^0
  wires:
  Gain/1 -> Delay1/1
  Minimum/1 -> Compare To Constant1/1
  Compare To Constant1/1 -> Add1/2
  Delay2/1 -> Add1/1, N/1
  Add1/1 -> Delay2/1
  Num/1 -> For Iterator/1
  Data Type  Conversion3/1 -> Reshape/1
  Compare To Constant/1 -> Switch1/2
  For Iterator/1 -> Compare To Constant/1, Assignment/2
  Switch1/1 -> Minimum/1
  Dis/1 -> Switch1/1, Assignment2/1, Assignment1/1
  Delay1/1 -> Switch1/3
  Assignment/1 -> Match/1
  Selector1/1 -> Assignment1/3
  Assignment1/1 -> Add/1
  Assignment2/1 -> Add/2
  Add/1 -> Gain/1
  Minimum/2 -> Data Type  Conversion3/1, Selector/1, Selector1/1
  Constant/1 -> Assignment1/2, Assignment2/2
  Selector/1 -> Assignment2/3
  Constant1/1 -> Matrix Concatenation1/1
  N1/1 -> Matrix Concatenation1/2
  N2/1 -> Matrix Concatenation1/3
  Matrix Concatenation1/1 -> Minimum/2
  Reshape/1 -> Assignment/1

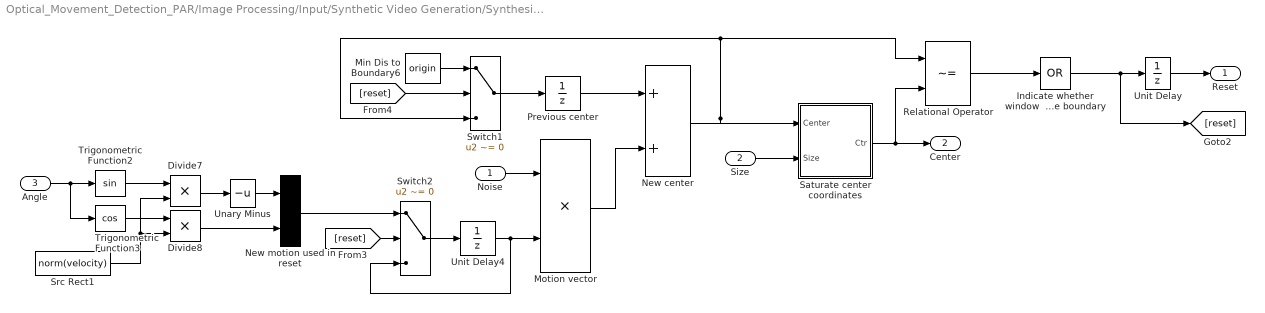
== system Optical_Movement_Detection_PAR/Image Processing/Input/Synthetic Video Generation/Synthesize Video/Center Locations ==
  Noise : Inport
  Size : Inport  Port=2  OutDataType=sfix(16)  OutScaling=2^0
  Angle : Inport  Port=3
  Divide7 : Product  Inputs=**  OutDataType=sfix(16)  OutScaling=2^-10
  Divide8 : Product  Inputs=**  OutDataType=sfix(16)  OutScaling=2^-10
  Indicate whether window  hit image boundary : Logic  Operator=OR  Inputs=1  AllPortsSameDT=off  OutDataTypeMode=boolean  OutDataTypeStr=boolean
  Min Dis to Boundary6 : Constant  Value=origin  OutDataType=sfix(16)  OutScaling=2^0
  Motion vector : Product  Inputs=**  OutDataType=sfix(16)  OutScaling=2^-10
  New center : Sum  OutDataType=sfix(16)  OutScaling=2^-10
  New motion used in reset : Concatenate  Mode=Vector
  Previous center : UnitDelay  X0=origin  SampleTime=-1
  Relational Operator : RelationalOperator  Operator=~=  LogicOutDataTypeMode=boolean  OutDataTypeStr=boolean
  Saturate center coordinates : Subsystem
  Src Rect1 : Constant  Value=norm(velocity)  VectorParams1D=off  OutDataType=sfix(16)  OutScaling=2^0  OutDataTypeStr=Inherit: Inherit via back propagation
  Switch1 : Switch  Criteria=u2 ~= 0  OutDataType=sfix(16)  OutScaling=2^0
  Switch2 : Switch  Criteria=u2 ~= 0  OutDataType=sfix(16)  OutScaling=2^0
  Trigonometric Function2 : Trigonometry
  Trigonometric Function3 : Trigonometry  Operator=cos
  Unary Minus : UnaryMinus
  Unit Delay : UnitDelay  X0=1  SampleTime=-1
  Unit Delay4 : UnitDelay  X0=velocity  SampleTime=-1
  Reset : Outport
  Center : Outport  Port=2
  wires:
  Unit Delay4/1 -> Switch2/3, Motion vector/2
  Previous center/1 -> New center/1
  [reset] -> Switch1/2
  [reset] -> Switch2/2
  Divide7/1 -> Unary Minus/1
  Unary Minus/1 -> New motion used in reset/1
  Divide8/1 -> New motion used in reset/2
  Src Rect1/1 -> Divide8/2, Divide7/2
  Switch1/1 -> Previous center/1
  Min Dis to Boundary6/1 -> Switch1/1
  Switch2/1 -> Unit Delay4/1
  New motion used in reset/1 -> Switch2/1
  Trigonometric Function3/1 -> Divide8/1
  Trigonometric Function2/1 -> Divide7/1
  Angle/1 -> Trigonometric Function3/1, Trigonometric Function2/1
  Relational Operator/1 -> Indicate whether window  hit image boundary/1
  Indicate whether window  hit image boundary/1 -> [reset], Unit Delay/1
  Saturate center coordinates/1(Ctr) -> Center/1, Relational Operator/2
  Size/1 -> Saturate center coordinates/2(Size)
  New center/1 -> Switch1/3, Relational Operator/1, Saturate center coordinates/1(Center)
  Unit Delay/1 -> Reset/1
  Motion vector/1 -> New center/2
  Noise/1 -> Motion vector/1

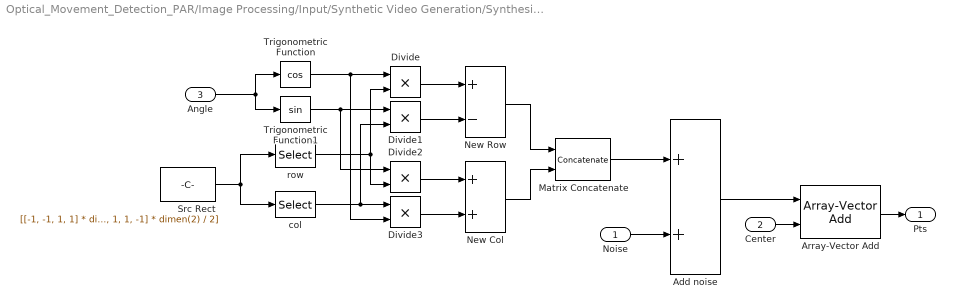
== system Optical_Movement_Detection_PAR/Image Processing/Input/Synthetic Video Generation/Synthesize Video/Corner Locations ==
  Noise : Inport
  Center : Inport  Port=2
  Angle : Inport  Port=3
  Add noise : Sum  OutDataType=sfix(16)  OutScaling=2^-10
  Array-Vector Add : dspmtrx3/Array-Vector Add  DialogController=dspDDGCreate  DialogControllerArgs=DataTag1  Dimension=1  V_Source=Input port  V_VectFromMask=[0.5 0.25]  firstCoeffDataTypeStr=Inherit: Same word length as input  firstCoeffLastDataTypeStr=Inherit: Same word length as input  firstCoeffMin=[]  firstCoeffMax=[]  outputDataTypeStr=Inherit: Same as accumulator  outputLastDataTypeStr=Inherit: Same as accumulator  outputMin=[]  outputMax=[]  roundingMode=Floor  overflowMode=off
  Divide{,1..3} (4 alike) : Product  Inputs=**  OutDataType=sfix(16)  OutScaling=2^-10
  Matrix Concatenate : Concatenate  Mode=Multidimensional array
  New Col : Sum  OutDataType=sfix(16)  OutScaling=2^-10
  New Row : Sum  Inputs=+-  OutDataType=sfix(16)  OutScaling=2^-10
  Src Rect : Constant  Value=[[-1, -1, 1, 1] * dimen(1) / 2; [-1, 1, 1, -1] * dimen(2) / 2]  OutDataType=sfix(16)  OutScaling=2^0
  Trigonometric Function : Trigonometry  Operator=cos
  Trigonometric Function1 : Trigonometry
  col : Selector  NumberOfDimensions=2  IndexMode=Zero-based  InputPortWidth=3  IndexOptions=Index vector (dialog),Select all  Indices=1,1  OutputSizes=1,1
  row : Selector  NumberOfDimensions=2  IndexMode=Zero-based  InputPortWidth=3  IndexOptions=Index vector (dialog),Select all  Indices=0,1  OutputSizes=1,1
  Pts : Outport
  wires:
  Noise/1 -> Add noise/2
  Center/1 -> Array-Vector Add/2
  Array-Vector Add/1 -> Pts/1
  Src Rect/1 -> col/1, row/1
  Divide2/1 -> New Col/1
  Divide3/1 -> New Col/2
  New Row/1 -> Matrix Concatenate/1
  New Col/1 -> Matrix Concatenate/2
  Matrix Concatenate/1 -> Add noise/1
  Angle/1 -> Trigonometric Function/1, Trigonometric Function1/1
  Divide/1 -> New Row/1
  Divide1/1 -> New Row/2
  Trigonometric Function/1 -> Divide3/2, Divide/1
  Trigonometric Function1/1 -> Divide2/1, Divide1/1
  row/1 -> Divide2/2, Divide/2
  col/1 -> Divide1/2, Divide3/1
  Add noise/1 -> Array-Vector Add/1

== system Optical_Movement_Detection_PAR/Image Processing/Optical Flow/Corner Matching/Calculate Distances/For Iterator Subsystem ==
  F1 : Inport  OutDataType=sfix(16)  OutScaling=2^0
  N1 : Inport  Port=2  OutDataType=sfix(16)  OutScaling=2^0
  F2 : Inport  Port=3  OutDataType=sfix(16)  OutScaling=2^0
  N2 : Inport  Port=4  OutDataType=sfix(16)  OutScaling=2^0
  For Iterator : ForIterator  IterationSource=external  IndexMode=Zero-based
  For Iterator Subsystem : Subsystem  TreatAsAtomicUnit=on
  Select feature  for 1 corner : Selector  NumberOfDimensions=2  IndexMode=Zero-based  InputPortWidth=2  IndexOptions=Select all,Index vector (port)  Indices=0,1  OutputSizes=1,1
  Update feature  for a corner : Assignment  NumberOfDimensions=2  IndexMode=Zero-based  OutputInitialize=Specify size for each dimension in table  IndexOptions=Assign all,Index vector (port)  Indices=1,1  OutputSizes=maxNum,maxNum
  Dis : Outport  OutDataType=sfix(16)  OutScaling=2^0
  wires:
  Update feature  for a corner/1 -> Dis/1
  N1/1 -> For Iterator Subsystem/2(N1)
  F1/1 -> For Iterator Subsystem/1(F1)
  Select feature  for 1 corner/1 -> For Iterator Subsystem/3(f2)
  F2/1 -> Select feature  for 1 corner/1
  For Iterator/1 -> Select feature  for 1 corner/2, Update feature  for a corner/2
  N2/1 -> For Iterator/1
  For Iterator Subsystem/1(Dis) -> Update feature  for a corner/1

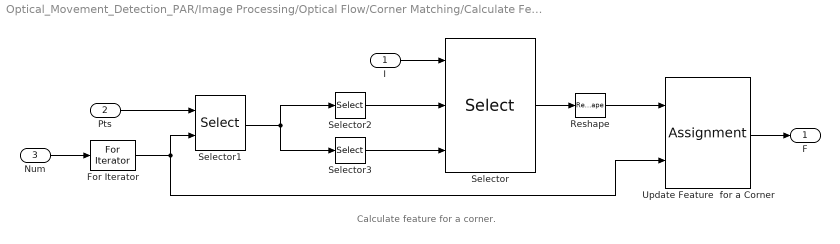
== system Optical_Movement_Detection_PAR/Image Processing/Optical Flow/Corner Matching/Calculate Features/Calculate Point Features ==
  note: Calculate feature for a corner.
  I : Inport
  Pts : Inport  Port=2
  Num : Inport  Port=3
  For Iterator : ForIterator  IterationSource=external  IndexMode=Zero-based
  Reshape : Reshape  OutputDimensionality=Column vector (2-D)
  Selector : Selector  NumberOfDimensions=2  IndexMode=Zero-based  InputPortWidth=3  IndexOptions=Starting index (port),Starting index (port)  Indices=[1 3],1  OutputSizes=winLen,winLen
  Selector1 : Selector  NumberOfDimensions=2  IndexMode=Zero-based  InputPortWidth=3  IndexOptions=Select all,Index vector (port)  Indices=[1 3],1  OutputSizes=9,9
  Selector2 : Selector  IndexMode=Zero-based  InputPortWidth=2  IndexOptions=Index vector (dialog)  Indices=0  OutputSizes=9
  Selector3 : Selector  IndexMode=Zero-based  InputPortWidth=2  IndexOptions=Index vector (dialog)  Indices=1  OutputSizes=9
  Update Feature  for a Corner : Assignment  NumberOfDimensions=2  IndexMode=Zero-based  OutputInitialize=Specify size for each dimension in table  IndexOptions=Assign all,Index vector (port)  Indices=1,1  OutputSizes=winLen^2,maxNum
  F : Outport
  wires:
  Selector3/1 -> Selector/3
  Selector2/1 -> Selector/2
  Num/1 -> For Iterator/1
  Update Feature  for a Corner/1 -> F/1
  Pts/1 -> Selector1/1
  I/1 -> Selector/1
  Reshape/1 -> Update Feature  for a Corner/1
  Selector/1 -> Reshape/1
  Selector1/1 -> Selector2/1, Selector3/1
  For Iterator/1 -> Update Feature  for a Corner/2, Selector1/2

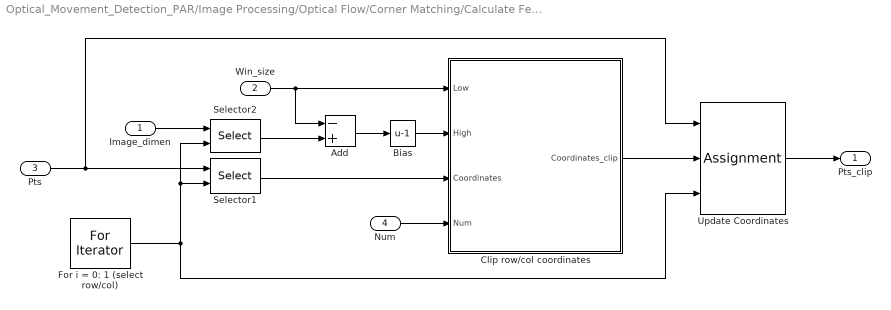
== system Optical_Movement_Detection_PAR/Image Processing/Optical Flow/Corner Matching/Calculate Features/Clip Point Coordinates ==
  Image_dimen : Inport  OutDataType=sfix(16)  OutScaling=2^0
  Win_size : Inport  Port=2  OutDataType=sfix(16)  OutScaling=2^0
  Pts : Inport  Port=3
  Num : Inport  Port=4
  Add : Sum  Inputs=-+  OutDataType=sfix(16)  OutScaling=2^-10
  Bias : Bias  Bias=-1
  Clip row/col coordinates : Subsystem
  For i = 0: 1 (select row/col) : ForIterator  IterationLimit=2  IndexMode=Zero-based
  Selector1 : Selector  NumberOfDimensions=2  IndexMode=Zero-based  InputPortWidth=3  IndexOptions=Index vector (port),Select all  Indices=[1 3],1  OutputSizes=9,9
  Selector2 : Selector  IndexMode=Zero-based  InputPortWidth=2  IndexOptions=Index vector (port)  Indices=[1 3]  OutputSizes=9
  Update Coordinates : Assignment  NumberOfDimensions=2  IndexMode=Zero-based  IndexOptions=Index vector (port),Assign all  Indices=1,1  OutputSizes=81,50
  Pts_clip : Outport  OutDataType=sfix(16)  OutScaling=2^0
  wires:
  Selector2/1 -> Add/2
  For i = 0: 1 (select row/col)/1 -> Selector1/2, Selector2/2, Update Coordinates/3
  Clip row/col coordinates/1(Coordinates_clip) -> Update Coordinates/2
  Bias/1 -> Clip row/col coordinates/2(High)
  Update Coordinates/1 -> Pts_clip/1
  Num/1 -> Clip row/col coordinates/4(Num)
  Selector1/1 -> Clip row/col coordinates/3(Coordinates)
  Win_size/1 -> Add/1, Clip row/col coordinates/1(Low)
  Add/1 -> Bias/1
  Image_dimen/1 -> Selector2/1
  Pts/1 -> Update Coordinates/1, Selector1/1

== system Optical_Movement_Detection_PAR/Image Processing/Input/Synthetic Video Generation/Synthesize Video/Center Locations/Saturate center coordinates ==
  Center : Inport
  Size : Inport  Port=2
  Center2 : Sum  Inputs=-+  OutDataType=sfix(16)  OutScaling=2^-10
  Min Dis to Boundary : Constant  Value=kron([ceil(sqrt(dimen(1)^2+dimen(2)^2)/2)], [1; 1])  OutDataType=sfix(16)  OutScaling=2^0
  MinMax : MinMax  Function=max  Inputs=2  OutDataType=sfix(16)  OutScaling=2^0
  MinMax1 : MinMax  Inputs=2  OutDataType=sfix(16)  OutScaling=2^0
  row1 : Selector  IndexMode=Zero-based  InputPortWidth=3  IndexOptions=Index vector (dialog)  Indices=[0 1]  OutputSizes=1
  Ctr : Outport
  wires:
  Size/1 -> row1/1
  MinMax1/1 -> Ctr/1
  Center/1 -> MinMax/1
  Center2/1 -> MinMax1/2
  MinMax/1 -> MinMax1/1
  row1/1 -> Center2/2
  Min Dis to Boundary/1 -> Center2/1, MinMax/2
